simulink model "questao4"  (R2023a)
settings: Solver=FixedStepAuto  StartTime=0.0  StopTime=100  FixedStep=1  RelTol=1e-3
settings Model: Creator=franz  LastModifiedBy=franz

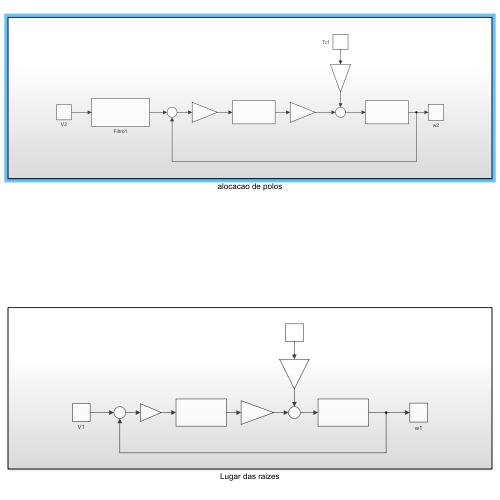
[thumbnail: Simulink's stored preview of the top-level diagram]
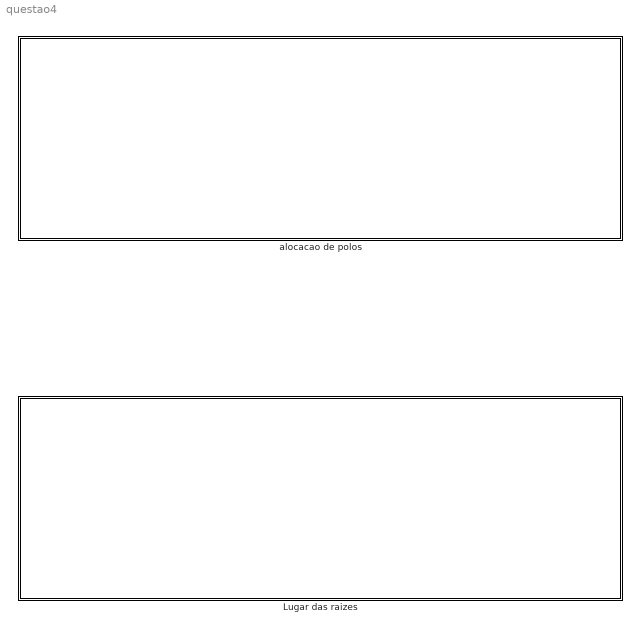
== system questao4 ==
  Lugar das raizes : Subsystem
  alocacao de polos : Subsystem

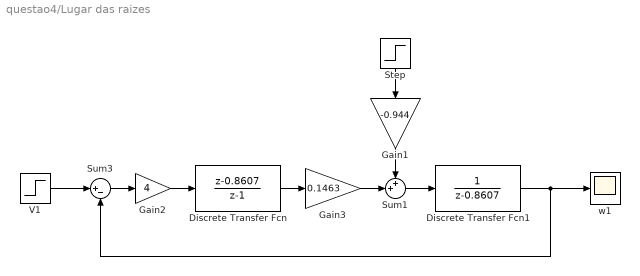
== system questao4/Lugar das raizes ==
  Discrete Transfer Fcn : DiscreteTransferFcn  Numerator=[1 -0.8607]  Denominator=[1 -1]
  Discrete Transfer Fcn1 : DiscreteTransferFcn  Numerator=[0 1]  Denominator=[1 -0.8607]
  Gain1 : Gain  Gain=-0.944
  Gain2 : Gain  Gain=4
  Gain3 : Gain  Gain=0.1463
  Step : Step  Time=30  After=0.25  SampleTime=0
  Sum1 : Sum  Inputs=++|
  Sum3 : Sum  Inputs=|+-
  V1 : Step  Time=10  SampleTime=0
  w1 : Scope
  wires:
  Sum3/1 -> Gain2/1
  Gain2/1 -> Discrete Transfer Fcn/1
  Discrete Transfer Fcn1/1 -> w1/1, Sum3/2
  V1/1 -> Sum3/1
  Discrete Transfer Fcn/1 -> Gain3/1
  Sum1/1 -> Discrete Transfer Fcn1/1
  Step/1 -> Gain1/1
  Gain1/1 -> Sum1/1
  Gain3/1 -> Sum1/2

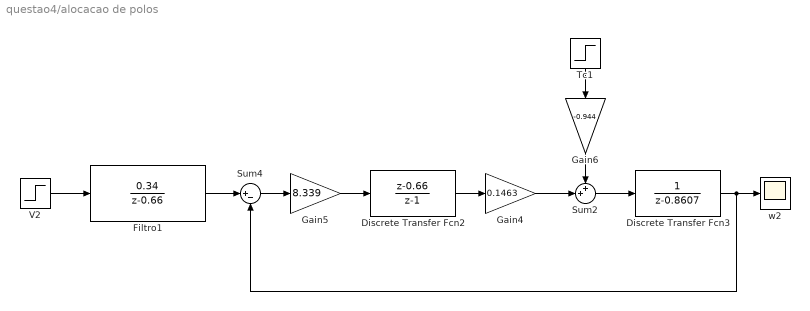
== system questao4/alocacao de polos ==
  Discrete Transfer Fcn2 : DiscreteTransferFcn  Numerator=[1 -0.66]  Denominator=[1 -1]
  Discrete Transfer Fcn3 : DiscreteTransferFcn  Numerator=[0 1]  Denominator=[1 -0.8607]
  Filtro1 : DiscreteTransferFcn  Numerator=[0 0.34]  Denominator=[1 -0.66]
  Gain4 : Gain  Gain=0.1463
  Gain5 : Gain  Gain=8.339
  Gain6 : Gain  Gain=-0.944
  Sum2 : Sum  Inputs=++|
  Sum4 : Sum  Inputs=|+-
  Tc1 : Step  Time=30  After=0.25  SampleTime=0
  V2 : Step  Time=10  SampleTime=0
  w2 : Scope
  wires:
  Filtro1/1 -> Sum4/1
  V2/1 -> Filtro1/1
  Sum2/1 -> Discrete Transfer Fcn3/1
  Gain5/1 -> Discrete Transfer Fcn2/1
  Discrete Transfer Fcn3/1 -> Sum4/2, w2/1
  Gain4/1 -> Sum2/2
  Gain6/1 -> Sum2/1
  Discrete Transfer Fcn2/1 -> Gain4/1
  Tc1/1 -> Gain6/1
  Sum4/1 -> Gain5/1
